simulink model "Nanogrid"  (R2026a)
settings: Solver=VariableStepAuto  StopTime=3
PreLoadFcn:
  | NanogridParam
undefined symbols (not defined in the file): baseLoad, bessSystem, bessVoltage, DiscIntNeverNeededParam, ee_sli_rtmsupport, gcbh, gflInverter, gfmInverter, nanoLoad, PV, PVInverter, ref, solar, solarInsolationChange, Ts
libraries: nesl_utility x51, eeGeneralControl x38, ee_lib x33, fl_lib x24, simulink x20, eeTransforms x13, slpidlib x8, nesl_utility_internal x4, sl_signal_attributes x4, sl_discontinuities x4, eeSinusoidalMeasurementV2 x3, batteryecm_lib x2
(part 6 of 6)

== system Nanogrid/Solar Plant Integrated/Detailed/PV Plant & Controller/Controller/MPPT/Solar PV Controller/Variant Subsystem/P&O MPP ==
  Ipv : Inport
  Vpv : Inport  Port=2
  AND1 : Logic  IconShape=distinctive  AllPortsSameDT=off  OutDataTypeStr=boolean
  Add : Sum
  Compare To Zero1 : simulink/Logic and Bit Operations/Compare To Zero  relop=>=  OutDataTypeStr=boolean
  Compare To Zero2 : simulink/Logic and Bit Operations/Compare To Zero  relop=>=  OutDataTypeStr=boolean
  Constant1 : Constant  Value=delV  SampleTime=sampleTime
  Data Type Conversion Inherited : sl_signal_attributes/Data Type Conversion Inherited  ConvertRealWorld=Real World Value  DoSatur=off
  Data Type Conversion Inherited1 : sl_signal_attributes/Data Type Conversion Inherited  ConvertRealWorld=Real World Value  DoSatur=off
  Filtered Derivative (Discrete or Continuous) : eeGeneralControl/Filtered Derivative (Discrete or Continuous)  K=1  T=tSettling*2  B=inf  A=-inf  minRatio=1  init_option=Inherited from block input  x0=0  Ts=sampleTime
  Filtered Derivative (Discrete or Continuous)1 : eeGeneralControl/Filtered Derivative (Discrete or Continuous)  K=1  T=tSettling*2  B=inf  A=-inf  minRatio=1  init_option=Inherited from block input  x0=0  Ts=sampleTime
  NOR : Logic  Operator=NOR  IconShape=distinctive  AllPortsSameDT=off  OutDataTypeStr=boolean
  OR : Logic  Operator=OR  IconShape=distinctive  AllPortsSameDT=off  OutDataTypeStr=boolean
  Product : Product
  Subtract5 : Sum  Inputs=-+
  Switch4 : Switch  Criteria=u2 ~= 0  SaturateOnIntegerOverflow=off  InputSameDT=off
  Switch5 : Switch  Criteria=u2 > Threshold  SaturateOnIntegerOverflow=off  InputSameDT=off
  start MPPT Voltage : Constant  Value=Vdc  SampleTime=sampleTime
  Vmpp : Outport  VectorParamsAs1DForOutWhenUnconnected=off
  wires:
  Data Type Conversion Inherited1/1 -> Subtract5/1, Add/2
  start MPPT Voltage/1 -> Data Type Conversion Inherited/2
  Data Type Conversion Inherited/1 -> Switch5/3
  Switch4/1 -> Vmpp/1
  Product/1 -> Filtered Derivative (Discrete or Continuous)/1
  Ipv/1 -> Product/1
  [Vinc] -> Switch4/1
  AND1/1 -> OR/1
  Filtered Derivative (Discrete or Continuous)/1 -> Compare To Zero2/1
  Filtered Derivative (Discrete or Continuous)1/1 -> Compare To Zero1/1
  [Vdec] -> Switch4/3
  Subtract5/1 -> [Vdec]  "DEC"
  NOR/1 -> OR/2
  Add/1 -> [Vinc]  "INC"
  Vpv/1 -> Switch5/1, Switch5/2, Data Type Conversion Inherited/1, Filtered Derivative (Discrete or Continuous)1/1, Product/2
  Constant1/1 -> Data Type Conversion Inherited1/2
  Switch5/1 -> Subtract5/2, Add/1, Data Type Conversion Inherited1/1
  Compare To Zero2/1 -> AND1/1, NOR/2
  Compare To Zero1/1 -> AND1/2, NOR/1
  OR/1 -> Switch4/2

== system Nanogrid/Solar Plant Integrated/Detailed/PV Plant & Controller/Controller/Power Reference/Power Reference Controller/PLL & Measurements/Measurement1 ==
  u : Inport
  Lead-Lag (Discrete or Continuous) : eeGeneralControl/Lead-Lag (Discrete or Continuous)  T1=0  T2=1e-3  B=inf  A=-inf  init_option=Inherited from block input  x0=0  Ts=Ts
  Vg : Outport
  wires:
  u/1 -> Lead-Lag (Discrete or Continuous)/1
  Lead-Lag (Discrete or Continuous)/1 -> Vg/1

== system Nanogrid/Solar Plant Integrated/Detailed/PV Plant & Controller/Controller/Power Reference/Power Reference Controller/PLL & Measurements/Measurement2 ==
  u : Inport
  Lead-Lag (Discrete or Continuous) : eeGeneralControl/Lead-Lag (Discrete or Continuous)  T1=0  T2=1e-3  B=inf  A=-inf  init_option=Inherited from block input  x0=0  Ts=Ts
  Vg : Outport
  wires:
  u/1 -> Lead-Lag (Discrete or Continuous)/1
  Lead-Lag (Discrete or Continuous)/1 -> Vg/1

== system Nanogrid/Solar Plant Integrated/Detailed/PV Plant & Controller/Controller/Power Reference/Power Reference Controller/PLL & Measurements/Subsystem ==
  Vabc : Inport
  Iabc : Inport  Port=2
  Demux : Demux  Outputs=3
  Demux1 : Demux  Outputs=3
  Park Transform : eeTransforms/Park Transform  AxisAlignment=Q-axis  PowerInvariant=off
  Park Transform1 : eeTransforms/Park Transform  AxisAlignment=Q-axis  PowerInvariant=off
  Scope : Scope  NumInputPorts=2
      settings: ActiveDisplayYMinimum=0.97158  ActiveDisplayYMaximum=1.00612  DataLoggingVariableName=ScopeData5
  "Sinusoidal Measurement (PLL, Three-Phase)" : eeSinusoidalMeasurementV2/Sinusoidal Measurement (PLL, Three-Phase)  InputFilter=on  InputNormalization=off  Kp_LF=kpPLL  Ki_LF=kiPLL  F0=frequency  Theta0=0  Ts=-1
  Terminator : Terminator
  Terminator1 : Terminator
  mag : Outport
  freq : Outport  Port=2
  angle : Outport  Port=3
  Vd : Outport  Port=4
  Vq : Outport  Port=5
  Id1 : Outport  Port=6
  Iq1 : Outport  Port=7
  wires:
  Iabc/1 -> Park Transform1/1
  Demux1/3 -> Terminator1/1
  Demux1/2 -> Iq1/1
  Demux1/1 -> Id1/1
  Park Transform1/1 -> Demux1/1
  "Sinusoidal Measurement (PLL, Three-Phase)"/3 -> mag/1
  "Sinusoidal Measurement (PLL, Three-Phase)"/1 -> freq/1
  "Sinusoidal Measurement (PLL, Three-Phase)"/2 -> Park Transform/2, Park Transform1/2, angle/1
  Demux/2 -> Vq/1, Scope/2
  Demux/1 -> Vd/1, Scope/1
  Park Transform/1 -> Demux/1
  Vabc/1 -> "Sinusoidal Measurement (PLL, Three-Phase)"/1, Park Transform/1
  Demux/3 -> Terminator/1

== system Nanogrid/Solar Plant Integrated/Detailed/PV Plant & Controller/Controller/Power Reference/Power Reference Controller/Power Reference Controller/Current_controller ==
  id-ref : Inport
  ipvd : Inport  Port=2
  iqref : Inport  Port=3
  iq : Inport  Port=4
  Vd : Inport  Port=5
  Vq : Inport  Port=6
  Constant4 : Constant  Value=0
  Gain1 : Gain  Gain=2*1*pi*60*L/zbase
  Gain2 : Gain  Gain=2*1*pi*60*L/zbase
  Mux1 : Mux  Inputs=3
  PID Controller : slpidlib/PID Controller  Controller=PID  Form=Parallel  TimeDomain=Discrete-time  UseExternalTs=off  SampleTime=-1  IntegratorMethod=Forward Euler  FilterMethod=Forward Euler  ControllerParametersSource=internal  P=Kpic  I=Kiic  UseKiTs=off  D=Kd  UseExternalDerivativeSource=off  N=100  UseFilter=on  TunerSelectOption=Transfer Function Based (PID Tuner App)  InitialConditionSource=internal  InitialConditionForIntegrator=0  InitialConditionForFilter=0  DifferentiatorICPrevScaledInput=0  ExternalReset=none  TrackingMode=off  Kt=1  LimitOutput=on  SatLimitsSource=internal  UpperSaturationLimit=3  LowerSaturationLimit=-3  LinearizeAsGain=on  AntiWindupMode=clamping  Kb=1  LimitIntegrator=on  UpperIntegratorSaturationLimit=3  LowerIntegratorSaturationLimit=-3  POutMin=[]  POutMax=[]  IOutMin=[]  IOutMax=[]  DOutMin=[]  DOutMax=[]  NOutMin=[]  NOutMax=[]  SumOutMin=[]  SumOutMax=[]  SaturationOutMin=[]  SaturationOutMax=[]  PParamMin=[]  PParamMax=[]  IParamMin=[]  IParamMax=[]  DParamMin=[]  DParamMax=[]  NParamMin=[]  NParamMax=[]  KbParamMin=[]  KbParamMax=[]  KtParamMin=[]  KtParamMax=[]  KbOutMin=[]  KbOutMax=[]  KtOutMin=[]  KtOutMax=[]  IntegratorOutMin=[]  IntegratorOutMax=[]  FilterOutMin=[]  FilterOutMax=[]  SumI1OutMin=[]  SumI1OutMax=[]  SumI2OutMin=[]  SumI2OutMax=[]  SumI3OutMin=[]  SumI3OutMax=[]  SumI4OutMin=[]  SumI4OutMax=[]  SumDOutMin=[]  SumDOutMax=[]  DifferentiatorOutMin=[]  DifferentiatorOutMax=[]  FilterDiffOutCoefMin=[]  FilterDiffOutCoefMax=[]  ReciprocalOutMin=[]  ReciprocalOutMax=[]  SumDenOutMin=[]  SumDenOutMax=[]  SumNumOutMin=[]  SumNumOutMax=[]  DivideOutMin=[]  DivideOutMax=[]  UdiffTsProdOutMin=[]  UdiffTsProdOutMax=[]  NTsProdOutMin=[]  NTsProdOutMax=[]  UintegralTsProdOutMin=[]  UintegralTsProdOutMax=[]  UngainTsProdOutMin=[]  UngainTsProdOutMax=[]  ClampingZeroOutDataTypeStr=Inherit: Inherit via back propagation  ClampingZeroOutMin=[]  ClampingZeroOutMax=[]  FilterDenConstantOutDataTypeStr=Inherit: Inherit via back propagation  FilterDenConstantOutMin=[]  FilterDenConstantOutMax=[]  PCopyOutDataTypeStr=Inherit: Inherit via back propagation  PCopyOutMin=[]  PCopyOutMax=[]  NCopyOutDataTypeStr=Inherit: Inherit via back propagation  NCopyOutMin=[]  NCopyOutMax=[]  IntegratorContinuousStateAttributes=''  IntegratorStateMustResolveToSignalObject=off  IntegratorRTWStateStorageClass=Auto  FilterContinuousStateAttributes=''  FilterStateMustResolveToSignalObject=off  FilterRTWStateStorageClass=Auto  ParallelPVariant=InternalParameters  IdealPVariant=Disabled  IVariant=InternalParameters  DVariant=InternalParameters  IntegratorVariant=Discrete  SatVariant=Enabled  AWVariant=DiscClampingParallel  PCopyVariant=Disabled  TRVariant=Disabled  FdbkBlocksVariant=Forward  IdealPFdbkVariant=Disabled  SatFdbkVariant=Disabled  DerivativeFilterVariant=ForwardEulerFilter  NVariant=InternalParameters  NCopyVariant=Disabled  FilterICVariant=InternalICsFilter  IntegratorICVariant=InternalICs  ExternalResetVariant=Disabled  TRSumVariant=Passthrough  SumFdbkVariant=Disabled  SumVariant=Sum_PID  TsampFilterVariant=InternalTs  TsampNgainVariant=Passthrough  TsampIntegralVariant=Disabled_SignalSpec  ExternalSaturationOutDataTypeStr=Inherit: Same as second input  DerivativeSourceVariant=ErrorSignal  PreIntVariant=InternalPreInt
  PID Controller1 : slpidlib/PID Controller  Controller=PID  Form=Parallel  TimeDomain=Discrete-time  UseExternalTs=off  SampleTime=-1  IntegratorMethod=Forward Euler  FilterMethod=Forward Euler  ControllerParametersSource=internal  P=Kpic  I=Kiic  UseKiTs=off  D=Kd  UseExternalDerivativeSource=off  N=100  UseFilter=on  TunerSelectOption=Transfer Function Based (PID Tuner App)  InitialConditionSource=internal  InitialConditionForIntegrator=0  InitialConditionForFilter=0  DifferentiatorICPrevScaledInput=0  ExternalReset=none  TrackingMode=off  Kt=1  LimitOutput=on  SatLimitsSource=internal  UpperSaturationLimit=3  LowerSaturationLimit=-3  LinearizeAsGain=on  AntiWindupMode=clamping  Kb=1  LimitIntegrator=on  UpperIntegratorSaturationLimit=3  LowerIntegratorSaturationLimit=-3  POutMin=[]  POutMax=[]  IOutMin=[]  IOutMax=[]  DOutMin=[]  DOutMax=[]  NOutMin=[]  NOutMax=[]  SumOutMin=[]  SumOutMax=[]  SaturationOutMin=[]  SaturationOutMax=[]  PParamMin=[]  PParamMax=[]  IParamMin=[]  IParamMax=[]  DParamMin=[]  DParamMax=[]  NParamMin=[]  NParamMax=[]  KbParamMin=[]  KbParamMax=[]  KtParamMin=[]  KtParamMax=[]  KbOutMin=[]  KbOutMax=[]  KtOutMin=[]  KtOutMax=[]  IntegratorOutMin=[]  IntegratorOutMax=[]  FilterOutMin=[]  FilterOutMax=[]  SumI1OutMin=[]  SumI1OutMax=[]  SumI2OutMin=[]  SumI2OutMax=[]  SumI3OutMin=[]  SumI3OutMax=[]  SumI4OutMin=[]  SumI4OutMax=[]  SumDOutMin=[]  SumDOutMax=[]  DifferentiatorOutMin=[]  DifferentiatorOutMax=[]  FilterDiffOutCoefMin=[]  FilterDiffOutCoefMax=[]  ReciprocalOutMin=[]  ReciprocalOutMax=[]  SumDenOutMin=[]  SumDenOutMax=[]  SumNumOutMin=[]  SumNumOutMax=[]  DivideOutMin=[]  DivideOutMax=[]  UdiffTsProdOutMin=[]  UdiffTsProdOutMax=[]  NTsProdOutMin=[]  NTsProdOutMax=[]  UintegralTsProdOutMin=[]  UintegralTsProdOutMax=[]  UngainTsProdOutMin=[]  UngainTsProdOutMax=[]  ClampingZeroOutDataTypeStr=Inherit: Inherit via back propagation  ClampingZeroOutMin=[]  ClampingZeroOutMax=[]  FilterDenConstantOutDataTypeStr=Inherit: Inherit via back propagation  FilterDenConstantOutMin=[]  FilterDenConstantOutMax=[]  PCopyOutDataTypeStr=Inherit: Inherit via back propagation  PCopyOutMin=[]  PCopyOutMax=[]  NCopyOutDataTypeStr=Inherit: Inherit via back propagation  NCopyOutMin=[]  NCopyOutMax=[]  IntegratorContinuousStateAttributes=''  IntegratorStateMustResolveToSignalObject=off  IntegratorRTWStateStorageClass=Auto  FilterContinuousStateAttributes=''  FilterStateMustResolveToSignalObject=off  FilterRTWStateStorageClass=Auto  ParallelPVariant=InternalParameters  IdealPVariant=Disabled  IVariant=InternalParameters  DVariant=InternalParameters  IntegratorVariant=Discrete  SatVariant=Enabled  AWVariant=DiscClampingParallel  PCopyVariant=Disabled  TRVariant=Disabled  FdbkBlocksVariant=Forward  IdealPFdbkVariant=Disabled  SatFdbkVariant=Disabled  DerivativeFilterVariant=ForwardEulerFilter  NVariant=InternalParameters  NCopyVariant=Disabled  FilterICVariant=InternalICsFilter  IntegratorICVariant=InternalICs  ExternalResetVariant=Disabled  TRSumVariant=Passthrough  SumFdbkVariant=Disabled  SumVariant=Sum_PID  TsampFilterVariant=InternalTs  TsampNgainVariant=Passthrough  TsampIntegralVariant=Disabled_SignalSpec  ExternalSaturationOutDataTypeStr=Inherit: Same as second input  DerivativeSourceVariant=ErrorSignal  PreIntVariant=InternalPreInt
  Saturation : Saturate  UpperLimit=1.2  LowerLimit=-1.2
  Saturation1 : Saturate  UpperLimit=1.2  LowerLimit=-1.2
  Scope : Scope  NumInputPorts=2
      settings: ActiveDisplayYMinimum=0.49995  ActiveDisplayYMaximum=0.50039
  Scope1 : Scope  NumInputPorts=2
      settings: ActiveDisplayYMinimum=-1  ActiveDisplayYMaximum=1  DataLoggingVariableName=ScopeData2
  Scope2 : Scope  NumInputPorts=3
      settings: ActiveDisplayYMinimum=0.92426  ActiveDisplayYMaximum=1.0261  DataLoggingVariableName=ScopeData2
  Sum1 : Sum  Inputs=|+-
  Sum3 : Sum  Inputs=|++-
  Sum4 : Sum  Inputs=|+++
  Sum5 : Sum  Inputs=|+-
  mdq0 : Outport
  wires:
  Vd/1 -> Sum3/1, Scope2/1
  Saturation1/1 -> Mux1/2
  Saturation/1 -> Mux1/1
  iqref/1 -> Sum5/1, Scope1/1
  Mux1/1 -> mdq0/1
  Sum4/1 -> [Eq], Saturation1/1
  PID Controller1/1 -> Sum4/1
  Sum5/1 -> PID Controller1/1
  Constant4/1 -> Mux1/3
  Sum1/1 -> PID Controller/1
  iq/1 -> Sum5/2, Gain2/1, Scope1/2
  Vq/1 -> Sum4/2
  Gain1/1 -> Sum4/3
  id-ref/1 -> Sum1/1, Scope/1
  ipvd/1 -> Sum1/2, Gain1/1, Scope/2
  Gain2/1 -> Sum3/3, Scope2/3
  Sum3/1 -> [Ed], Saturation/1
  PID Controller/1 -> Sum3/2, Scope2/2

== system Nanogrid/Solar Plant Integrated/Detailed/PV Plant & Controller/Controller/Power Reference/Power Reference Controller/Power Reference Controller/Reference Current ==
  note: Avoid division by zero during start
  note: Current Limiters
  V-mag : Inport
  LVRT_iq : Inport  Port=2
  PRef : Inport  Port=3
  QRef : Inport  Port=4
  Constant1 : Constant
  Constant3 : Constant  Value=Imax
  Current limits : Subsystem
  Refernce id generation : Subsystem
  Refernce iq generation : Subsystem
  Switch : Switch  Criteria=u2 ~= 0  SaturateOnIntegerOverflow=off  InputSameDT=off
  Unit Delay1 : UnitDelay  SampleTime=Ts
  Unit Delay3 : UnitDelay  SampleTime=Ts
  id_ref : Outport
  iq_ref : Outport  Port=2
  wires:
  Current limits/2(iubd) -> Refernce id generation/2(ubid)
  PRef/1 -> Refernce id generation/3(PRef)
  QRef/1 -> Refernce iq generation/4(Q_ref)
  Constant1/1 -> Switch/3
  Switch/1 -> Refernce iq generation/2(V_mag), Refernce id generation/1(V_mag)
  V-mag/1 -> Switch/2, Switch/1
  LVRT_iq/1 -> Refernce iq generation/3(LVRT_iq)
  Refernce iq generation/1(iq_ref) -> iq_ref/1, Unit Delay1/1
  Refernce id generation/1(id_ref) -> Unit Delay3/1, id_ref/1
  Constant3/1 -> Current limits/1(Imax)
  Unit Delay3/1 -> Current limits/3(idref)
  Current limits/1(iubq) -> Refernce iq generation/1(ubiq)
  Unit Delay1/1 -> Current limits/2(iqref)

== system Nanogrid/BESS Integrated/Detailed/BESS Controller/Grid Forming/Current Limiting/CurrentLimitingMethod/currentLimitAndVirtual/Current Saturation/Compare ==
  u : Inport
  Compare To Zero : simulink/Logic and Bit Operations/Compare To Zero  relop=<=  OutDataTypeStr=boolean
  Data Type Conversion : DataTypeConversion  SaturateOnIntegerOverflow=off  RndMeth=Floor
  Out1 : Outport
  wires:
  Data Type Conversion/1 -> Out1/1
  u/1 -> Compare To Zero/1
  Compare To Zero/1 -> Data Type Conversion/1

== system Nanogrid/BESS Integrated/Detailed/BESS Controller/Grid Forming/Current Limiting/CurrentLimitingMethod/currentLimitAndVirtual/Current Saturation/If Action Subsystem ==
  Is : Inport
  Isd : Inport  Port=2
  Isq : Inport  Port=3
  maxI : Inport  Port=4
  Action Port : ActionPort
  Divide : Product  Inputs=*/
  Product : Product
  Product1 : Product
  Idmax : Outport
  Iqmax : Outport  Port=2
  wires:
  Product/1 -> Iqmax/1
  Product1/1 -> Idmax/1
  Isq/1 -> Product/2
  Isd/1 -> Product1/1
  Divide/1 -> Product/1, Product1/2
  Is/1 -> Divide/2
  maxI/1 -> Divide/1

== system Nanogrid/BESS Integrated/Detailed/BESS Controller/Grid Forming/Current Limiting/CurrentLimitingMethod/currentLimitAndVirtual/Current Saturation/If Action Subsystem1 ==
  Action Port : ActionPort
  Constant3 : Constant  Value=0
  Constant4 : Constant  Value=0
  Idmax : Outport
  Iqmax : Outport  Port=2
  wires:
  Constant3/1 -> Idmax/1
  Constant4/1 -> Iqmax/1

== system Nanogrid/BESS Integrated/Detailed/BESS Controller/Grid Forming/Measurement/Frequency Measurement/Frequency Measurement/If Action Subsystem/Frequency estimation ==
  sk : Inport
  sk-1 : Inport  Port=2
  k : Inport  Port=3
  k-1 : Inport  Port=4
  Trigger : TriggerPort  VariantControl=(inherit)  InitialTriggerSignalState=positive
  Add1 : Sum  Inputs=+-  OutDataTypeStr=double  AccumDataTypeStr=double  RndMeth=Convergent
  Add2 : Sum
  Constant : Constant
  Delay : Delay  DelayLength=1
  Delay1 : Delay  DelayLength=1
  Divide : Product  Inputs=*/  RndMeth=Ceiling
  Gain : Gain  Gain=2  ParamDataTypeStr=double  RndMeth=Convergent
  Gain2 : Gain  Gain=0.5
  MATLAB Function : MATLAB Function  TreatAsAtomicUnit=on
  f : Outport
  wires:
  sk-1/1 -> MATLAB Function/2(y2)
  sk/1 -> MATLAB Function/1(y1)
  k-1/1 -> MATLAB Function/4(x2)  "x1"
  k/1 -> MATLAB Function/3(x1)
  Delay/1 -> Add1/2
  Gain2/1 -> f/1
  Add2/1 -> Gain2/1
  Delay1/1 -> Add2/2
  Divide/1 -> Delay1/1, Add2/1
  MATLAB Function/1(x) -> Add1/1, Delay/1  "x1-y1/slope"
  Gain/1 -> Divide/2
  Constant/1 -> Divide/1
  Add1/1 -> Gain/1

== system Nanogrid/BESS Integrated/Detailed/BESS Controller/Grid Forming/Power Control/ActivePowerControl/vsmControl/Damping Frequency/ConstantFreqReference ==
  fref : Inport
  Constant1 : Constant
  Terminator : Terminator
  fmeas : Outport
  wires:
  fref/1 -> Terminator/1
  Constant1/1 -> fmeas/1

== system Nanogrid/BESS Integrated/Detailed/BESS Controller/Grid Forming/Power Control/ActivePowerControl/vsmControl/Damping Frequency/WithFrequencyMeasurement ==
  fref : Inport
  fmeas : Outport
  wires:
  fref/1 -> fmeas/1

== system Nanogrid/BESS Integrated/Detailed/BESS Controller/Grid Forming/Power Control/ActivePowerControl/vsmControl/Power Reference Selection/If Action Subsystem ==
  note: Frequency difference power
  Pref : Inport
  Wsm : Inport  Port=2
  Action Port : ActionPort  ActionPortLabel=if(u1 > 0)
  Constant : Constant
  Gain6 : Gain  Gain=vsmFreqDroop
  Sum : Sum  Inputs=|+-
  Sum3 : Sum  Inputs=++|
  Power : Outport
  wires:
  Sum3/1 -> Power/1
  Constant/1 -> Sum/1
  Sum/1 -> Gain6/1
  Wsm/1 -> Sum/2
  Pref/1 -> Sum3/1  "Reference power"
  Gain6/1 -> Sum3/2

== system Nanogrid/BESS Integrated/Detailed/BESS Controller/Grid Forming/Power Control/ActivePowerControl/vsmControl/Power Reference Selection/If Action Subsystem1 ==
  note: Frequency difference power
  fref : Inport
  Wsm : Inport  Port=2
  Action Port : ActionPort  ActionPortLabel=else
  Gain6 : Gain  Gain=vsmFreqDroop
  Scope : Scope
      settings: ActiveDisplayYMinimum=0.99966  ActiveDisplayYMaximum=1.00057  DataLoggingVariableName=ScopeData14
  Scope1 : Scope
      settings: DataLoggingVariableName=ScopeData15
  Sum : Sum  Inputs=|+-
  Power : Outport
  wires:
  Gain6/1 -> Power/1, Scope1/1
  fref/1 -> Sum/1
  Sum/1 -> Gain6/1
  Wsm/1 -> Sum/2, Scope/1

== system Nanogrid/Solar Plant Integrated/Detailed/PV Plant & Controller/Controller/MPPT/Solar PV Controller/DC voltage controller & current reference/If Action Subsystem/Subsystem ==
  V mag : Inport
  iq ub : Inport  Port=2
  Q ref : Inport  Port=3
  Constant : Constant  Value=1e-3
  Data Type Conversion Inherited : simulink/Signal Attributes/Data Type Conversion Inherited  ConvertRealWorld=Real World Value  DoSatur=off
  Divide2 : Product  Inputs=*/
  Gain3 : Gain  Gain=-1
  Saturation Dynamic2 : simulink/Discontinuities/Saturation Dynamic  OutMin=[]  OutMax=[]  OutDataTypeStr=Inherit: Same as second input  OutDataType=fixdt(1, 16)  OutScaling=2^-10  DoSatur=off
  Switch : Switch  Criteria=u2 ~= 0  SaturateOnIntegerOverflow=off  InputSameDT=off
  iq ub1 : InportShadow  Port=2
  iqref : Outport
  wires:
  Data Type Conversion Inherited/1 -> Switch/3
  Constant/1 -> Data Type Conversion Inherited/2
  Switch/1 -> Divide2/2
  V mag/1 -> Switch/1, Switch/2, Data Type Conversion Inherited/1
  Saturation Dynamic2/1 -> iqref/1
  iq ub/1 -> Saturation Dynamic2/1
  Gain3/1 -> Saturation Dynamic2/3
  Q ref/1 -> Divide2/1
  Divide2/1 -> Saturation Dynamic2/2
  iq ub1/1 -> Gain3/1

== system Nanogrid/Solar Plant Integrated/Detailed/PV Plant & Controller/Controller/MPPT/Solar PV Controller/DC voltage controller & current reference/If Action Subsystem/Subsystem1 ==
  Vmag : Inport
  P pv : Inport  Port=2
  vdc : Inport  Port=3
  vdc ref : Inport  Port=4
  id ub : Inport  Port=5
  Constant : Constant  Value=1e-3
  Constant4 : Constant  Value=0
  Data Type Conversion Inherited : simulink/Signal Attributes/Data Type Conversion Inherited  ConvertRealWorld=Real World Value  DoSatur=off
  Divide : Product  Inputs=/*
  Gain4 : Gain  Gain=1/(mVAbase)
  Saturation Dynamic1 : simulink/Discontinuities/Saturation Dynamic  OutMin=[]  OutMax=[]  OutDataTypeStr=Inherit: Same as second input  OutDataType=fixdt(1, 16)  OutScaling=2^-10  DoSatur=off
  Scope : Scope  NumInputPorts=2
      settings: ActiveDisplayYMinimum=-55957.97767  ActiveDisplayYMaximum=503630.2665
  Sum : Sum  Inputs=|++
  Switch : Switch  Criteria=u2 ~= 0  SaturateOnIntegerOverflow=off  InputSameDT=off
  V_dc_Controller1 : Subsystem
  idref : Outport
  wires:
  Data Type Conversion Inherited/1 -> Switch/3
  Constant/1 -> Data Type Conversion Inherited/2
  Switch/1 -> Divide/1
  Vmag/1 -> Switch/1, Switch/2, Data Type Conversion Inherited/1
  vdc/1 -> Scope/1, V_dc_Controller1/1(vdc)
  Saturation Dynamic1/1 -> idref/1
  Divide/1 -> Sum/1
  Gain4/1 -> Divide/2
  id ub/1 -> Saturation Dynamic1/1
  vdc ref/1 -> Scope/2, V_dc_Controller1/2(vdc ref)
  Sum/1 -> Saturation Dynamic1/2
  V_dc_Controller1/1(Out1) -> Sum/2
  P pv/1 -> Gain4/1
  Constant4/1 -> Saturation Dynamic1/3

== system Nanogrid/Solar Plant Integrated/Detailed/PV Plant & Controller/Controller/MPPT/Solar PV Controller/DC voltage controller & current reference/Subsystem1/V_dc_Controller1 ==
  vdc : Inport
  vdc ref : Inport  Port=2
  Gain : Gain  Gain=1/VdcBase
  PID Controller : slpidlib/PID Controller  Controller=PID  Form=Parallel  TimeDomain=Discrete-time  UseExternalTs=off  SampleTime=-1  IntegratorMethod=Forward Euler  FilterMethod=Forward Euler  ControllerParametersSource=internal  P=Kpv  I=Kiv  UseKiTs=off  D=Kdv  UseExternalDerivativeSource=off  N=100  UseFilter=on  TunerSelectOption=Transfer Function Based (PID Tuner App)  ZeroCross=off  InitialConditionSource=internal  InitialConditionForIntegrator=0  InitialConditionForFilter=0  DifferentiatorICPrevScaledInput=0  ExternalReset=none  TrackingMode=off  Kt=1  LimitOutput=off  SatLimitsSource=internal  UpperSaturationLimit=iMax  LowerSaturationLimit=0  LinearizeAsGain=on  AntiWindupMode=clamping  Kb=1  LimitIntegrator=off  UpperIntegratorSaturationLimit=inf  LowerIntegratorSaturationLimit=-inf  POutMin=[]  POutMax=[]  IOutMin=[]  IOutMax=[]  DOutMin=[]  DOutMax=[]  NOutMin=[]  NOutMax=[]  SumOutMin=[]  SumOutMax=[]  SaturationOutMin=[]  SaturationOutMax=[]  PParamMin=[]  PParamMax=[]  IParamMin=[]  IParamMax=[]  DParamMin=[]  DParamMax=[]  NParamMin=[]  NParamMax=[]  KbParamMin=[]  KbParamMax=[]  KtParamMin=[]  KtParamMax=[]  KbOutMin=[]  KbOutMax=[]  KtOutMin=[]  KtOutMax=[]  IntegratorOutMin=[]  IntegratorOutMax=[]  FilterOutMin=[]  FilterOutMax=[]  SumI1OutMin=[]  SumI1OutMax=[]  SumI2OutMin=[]  SumI2OutMax=[]  SumI3OutMin=[]  SumI3OutMax=[]  SumI4OutMin=[]  SumI4OutMax=[]  SumDOutMin=[]  SumDOutMax=[]  DifferentiatorOutMin=[]  DifferentiatorOutMax=[]  FilterDiffOutCoefMin=[]  FilterDiffOutCoefMax=[]  ReciprocalOutMin=[]  ReciprocalOutMax=[]  SumDenOutMin=[]  SumDenOutMax=[]  SumNumOutMin=[]  SumNumOutMax=[]  DivideOutMin=[]  DivideOutMax=[]  UdiffTsProdOutMin=[]  UdiffTsProdOutMax=[]  NTsProdOutMin=[]  NTsProdOutMax=[]  UintegralTsProdOutMin=[]  UintegralTsProdOutMax=[]  UngainTsProdOutMin=[]  UngainTsProdOutMax=[]  ClampingZeroOutDataTypeStr=Inherit: Inherit via back propagation  ClampingZeroOutMin=[]  ClampingZeroOutMax=[]  FilterDenConstantOutDataTypeStr=Inherit: Inherit via back propagation  FilterDenConstantOutMin=[]  FilterDenConstantOutMax=[]  PCopyOutDataTypeStr=Inherit: Inherit via back propagation  PCopyOutMin=[]  PCopyOutMax=[]  NCopyOutDataTypeStr=Inherit: Inherit via back propagation  NCopyOutMin=[]  NCopyOutMax=[]  IntegratorContinuousStateAttributes=''  IntegratorStateMustResolveToSignalObject=off  IntegratorRTWStateStorageClass=Auto  FilterContinuousStateAttributes=''  FilterStateMustResolveToSignalObject=off  FilterRTWStateStorageClass=Auto  ParallelPVariant=InternalParameters  IdealPVariant=Disabled  IVariant=InternalParameters  DVariant=InternalParameters  IntegratorVariant=Discrete  SatVariant=Disabled  AWVariant=Passthrough  PCopyVariant=Disabled  TRVariant=Disabled  FdbkBlocksVariant=Forward  IdealPFdbkVariant=Disabled  SatFdbkVariant=Disabled  DerivativeFilterVariant=ForwardEulerFilter  NVariant=InternalParameters  NCopyVariant=Disabled  FilterICVariant=InternalICsFilter  IntegratorICVariant=InternalICs  ExternalResetVariant=Disabled  TRSumVariant=Passthrough  SumFdbkVariant=Disabled  SumVariant=Sum_PID  TsampFilterVariant=InternalTs  TsampNgainVariant=Passthrough  TsampIntegralVariant=Disabled_SignalSpec  ExternalSaturationOutDataTypeStr=Inherit: Same as second input  DerivativeSourceVariant=ErrorSignal  PreIntVariant=InternalPreInt
  Sum : Sum  Inputs=|+-
  Out1 : Outport
  wires:
  Sum/1 -> Gain/1
  Gain/1 -> PID Controller/1
  PID Controller/1 -> Out1/1
  vdc ref/1 -> Sum/2
  vdc/1 -> Sum/1

== system Nanogrid/Solar Plant Integrated/Detailed/PV Plant & Controller/Controller/Power Reference/Power Reference Controller/Power Reference Controller/Reference Current/Current limits ==
  Imax : Inport
  iqref : Inport  Port=2
  idref : Inport  Port=3
  Constant8 : Constant  Value=0
  Constant9 : Constant  Value=0
  Scope : Scope
      settings: ActiveDisplayYMinimum=-0.15  ActiveDisplayYMaximum=1.35  DataLoggingVariableName=ScopeData3
  Scope1 : Scope
      settings: ActiveDisplayYMinimum=-0.08298  ActiveDisplayYMaximum=0.74678  DataLoggingVariableName=ScopeData4
  Sqrt : Sqrt
  Sqrt1 : Sqrt
  Square{1..4} (4 alike) : Math  Operator=square
  Step2 : Step  Time=0.01  SampleTime=Ts
  Step3 : Step  Time=0.01  SampleTime=Ts
  Sum6 : Sum  Inputs=|+-
  Sum9 : Sum  Inputs=|+-
  Switch1 : Switch  Threshold=.01  SaturateOnIntegerOverflow=off  InputSameDT=off
  Switch2 : Switch  Threshold=.01  SaturateOnIntegerOverflow=off  InputSameDT=off
  iubq : Outport
  iubd : Outport  Port=2
  wires:
  idref/1 -> Square4/1
  Sqrt1/1 -> iubq/1, Scope1/1
  Imax/1 -> Square1/1, Square3/1
  Sqrt/1 -> iubd/1, Scope/1
  Constant9/1 -> Switch2/3
  Square4/1 -> Sum9/2
  Constant8/1 -> Switch1/3
  Square2/1 -> Sum6/2
  Sum6/1 -> Switch1/1
  Square3/1 -> Sum9/1
  iqref/1 -> Square2/1
  Switch1/1 -> Sqrt/1
  Square1/1 -> Sum6/1
  Switch2/1 -> Sqrt1/1
  Step2/1 -> Switch1/2
  Step3/1 -> Switch2/2
  Sum9/1 -> Switch2/1

== system Nanogrid/Solar Plant Integrated/Detailed/PV Plant & Controller/Controller/Power Reference/Power Reference Controller/Power Reference Controller/Reference Current/Refernce id generation ==
  V_mag : Inport
  ubid : Inport  Port=2
  PRef : Inport  Port=3
  Divide : Product  Inputs=/*
  Gain6 : Gain  Gain=-1
  P/Q Priority : Switch  Criteria=u2 ~= 0  SaturateOnIntegerOverflow=off  InputSameDT=off
  Priority Mode : Constant  Value=P-2
  Saturation Dynamic2 : sl_discontinuities/Saturation Dynamic  OutMin=[]  OutMax=[]  OutDataTypeStr=Inherit: Same as second input  OutDataType=fixdt(1, 16)  OutScaling=2^-10  DoSatur=off
  Saturation1 : Saturate  UpperLimit=Imax  LowerLimit=-Imax
  Scope : Scope
      settings: ActiveDisplayYMinimum=0.99583  ActiveDisplayYMaximum=1.02853
  Scope1 : Scope
      settings: ActiveDisplayYMinimum=-0.12499  ActiveDisplayYMaximum=1.12489  DataLoggingVariableName=ScopeData2
  ubid1 : InportShadow  Port=2
  id_ref : Outport
  wires:
  Divide/1 -> Saturation1/1, Saturation Dynamic2/2
  V_mag/1 -> Divide/1
  P/Q Priority/1 -> id_ref/1, Scope/1
  ubid1/1 -> Gain6/1
  Saturation1/1 -> P/Q Priority/1
  Priority Mode/1 -> P/Q Priority/2
  Saturation Dynamic2/1 -> P/Q Priority/3, Scope1/1
  Gain6/1 -> Saturation Dynamic2/3
  ubid/1 -> Saturation Dynamic2/1
  PRef/1 -> Divide/2

== system Nanogrid/Solar Plant Integrated/Detailed/PV Plant & Controller/Controller/Power Reference/Power Reference Controller/Power Reference Controller/Reference Current/Refernce iq generation ==
  ubiq : Inport
  V_mag : Inport  Port=2
  LVRT_iq : Inport  Port=3
  Q_ref : Inport  Port=4
  Divide1 : Product  Inputs=*/
  Gain : Gain  Gain=-1
  Gain1 : Gain  Gain=-1
  Gain7 : Gain  Gain=-1
  LVRT Priority : Switch  Threshold=.9  SaturateOnIntegerOverflow=off  InputSameDT=off
  P/Q Priority : Switch  Criteria=u2 ~= 0  SaturateOnIntegerOverflow=off  InputSameDT=off
  Priority Mode : Constant  Value=P-2
  Saturation Dynamic : sl_discontinuities/Saturation Dynamic  OutMin=[]  OutMax=[]  OutDataTypeStr=Inherit: Same as second input  OutDataType=fixdt(1, 16)  OutScaling=2^-10  DoSatur=off
  Saturation2 : Saturate  UpperLimit=1  LowerLimit=-1
  Saturation3 : Saturate  UpperLimit=Imax  LowerLimit=-Imax
  Scope : Scope  NumInputPorts=3
      settings: ActiveDisplayYMinimum=-0.025  ActiveDisplayYMaximum=0.22499  DataLoggingVariableName=ScopeData10
  ubiq1 : InportShadow
  iq_ref : Outport
  wires:
  Gain/1 -> iq_ref/1
  V_mag/1 -> Divide1/2, LVRT Priority/2
  Q_ref/1 -> Divide1/1
  ubiq1/1 -> Gain7/1
  LVRT_iq/1 -> Saturation2/1
  Gain7/1 -> Saturation Dynamic/3
  Saturation Dynamic/1 -> P/Q Priority/1
  Divide1/1 -> Saturation Dynamic/2, Saturation3/1
  Priority Mode/1 -> P/Q Priority/2
  Saturation3/1 -> P/Q Priority/3
  Saturation2/1 -> Gain1/1
  ubiq/1 -> Saturation Dynamic/1
  Gain1/1 -> LVRT Priority/3
  P/Q Priority/1 -> Scope/1, LVRT Priority/1
  LVRT Priority/1 -> Gain/1

== system Nanogrid/Solar Plant Integrated/Detailed/PV Plant & Controller/Controller/MPPT/Solar PV Controller/DC voltage controller & current reference/If Action Subsystem/Subsystem1/V_dc_Controller1 ==
  vdc : Inport
  vdc ref : Inport  Port=2
  Gain : Gain  Gain=1/VdcBase
  PID Controller : slpidlib/PID Controller  Controller=PID  Form=Parallel  TimeDomain=Discrete-time  UseExternalTs=off  SampleTime=-1  IntegratorMethod=Forward Euler  FilterMethod=Forward Euler  ControllerParametersSource=internal  P=Kpv  I=Kiv  UseKiTs=off  D=Kdv  UseExternalDerivativeSource=off  N=100  UseFilter=on  TunerSelectOption=Transfer Function Based (PID Tuner App)  ZeroCross=off  InitialConditionSource=internal  InitialConditionForIntegrator=0  InitialConditionForFilter=0  DifferentiatorICPrevScaledInput=0  ExternalReset=none  TrackingMode=off  Kt=1  LimitOutput=off  SatLimitsSource=internal  UpperSaturationLimit=iMax  LowerSaturationLimit=0  LinearizeAsGain=on  AntiWindupMode=clamping  Kb=1  LimitIntegrator=off  UpperIntegratorSaturationLimit=inf  LowerIntegratorSaturationLimit=-inf  POutMin=[]  POutMax=[]  IOutMin=[]  IOutMax=[]  DOutMin=[]  DOutMax=[]  NOutMin=[]  NOutMax=[]  SumOutMin=[]  SumOutMax=[]  SaturationOutMin=[]  SaturationOutMax=[]  PParamMin=[]  PParamMax=[]  IParamMin=[]  IParamMax=[]  DParamMin=[]  DParamMax=[]  NParamMin=[]  NParamMax=[]  KbParamMin=[]  KbParamMax=[]  KtParamMin=[]  KtParamMax=[]  KbOutMin=[]  KbOutMax=[]  KtOutMin=[]  KtOutMax=[]  IntegratorOutMin=[]  IntegratorOutMax=[]  FilterOutMin=[]  FilterOutMax=[]  SumI1OutMin=[]  SumI1OutMax=[]  SumI2OutMin=[]  SumI2OutMax=[]  SumI3OutMin=[]  SumI3OutMax=[]  SumI4OutMin=[]  SumI4OutMax=[]  SumDOutMin=[]  SumDOutMax=[]  DifferentiatorOutMin=[]  DifferentiatorOutMax=[]  FilterDiffOutCoefMin=[]  FilterDiffOutCoefMax=[]  ReciprocalOutMin=[]  ReciprocalOutMax=[]  SumDenOutMin=[]  SumDenOutMax=[]  SumNumOutMin=[]  SumNumOutMax=[]  DivideOutMin=[]  DivideOutMax=[]  UdiffTsProdOutMin=[]  UdiffTsProdOutMax=[]  NTsProdOutMin=[]  NTsProdOutMax=[]  UintegralTsProdOutMin=[]  UintegralTsProdOutMax=[]  UngainTsProdOutMin=[]  UngainTsProdOutMax=[]  ClampingZeroOutDataTypeStr=Inherit: Inherit via back propagation  ClampingZeroOutMin=[]  ClampingZeroOutMax=[]  FilterDenConstantOutDataTypeStr=Inherit: Inherit via back propagation  FilterDenConstantOutMin=[]  FilterDenConstantOutMax=[]  PCopyOutDataTypeStr=Inherit: Inherit via back propagation  PCopyOutMin=[]  PCopyOutMax=[]  NCopyOutDataTypeStr=Inherit: Inherit via back propagation  NCopyOutMin=[]  NCopyOutMax=[]  IntegratorContinuousStateAttributes=''  IntegratorStateMustResolveToSignalObject=off  IntegratorRTWStateStorageClass=Auto  FilterContinuousStateAttributes=''  FilterStateMustResolveToSignalObject=off  FilterRTWStateStorageClass=Auto  ParallelPVariant=InternalParameters  IdealPVariant=Disabled  IVariant=InternalParameters  DVariant=InternalParameters  IntegratorVariant=Discrete  SatVariant=Disabled  AWVariant=Passthrough  PCopyVariant=Disabled  TRVariant=Disabled  FdbkBlocksVariant=Forward  IdealPFdbkVariant=Disabled  SatFdbkVariant=Disabled  DerivativeFilterVariant=ForwardEulerFilter  NVariant=InternalParameters  NCopyVariant=Disabled  FilterICVariant=InternalICsFilter  IntegratorICVariant=InternalICs  ExternalResetVariant=Disabled  TRSumVariant=Passthrough  SumFdbkVariant=Disabled  SumVariant=Sum_PID  TsampFilterVariant=InternalTs  TsampNgainVariant=Passthrough  TsampIntegralVariant=Disabled_SignalSpec  ExternalSaturationOutDataTypeStr=Inherit: Same as second input  DerivativeSourceVariant=ErrorSignal  PreIntVariant=InternalPreInt
  Sum : Sum  Inputs=|+-
  Out1 : Outport
  wires:
  Sum/1 -> Gain/1
  Gain/1 -> PID Controller/1
  PID Controller/1 -> Out1/1
  vdc ref/1 -> Sum/2
  vdc/1 -> Sum/1

== stateflow chart Nanogrid/BESS Integrated/Detailed/BESS Controller/Grid Forming/Current Limiting/CurrentLimitingMethod/currentLimitAndVirtual/CurrentLimitSelection ==
  state Mode1_VI_ON
    entry:
    noCurrentLimit  = 0;
    viCurrentLimit = 1;
    satCurrentLimit = 0;
    ismax= maxVICurrentLimit;
    exit:
    noCurrentLimit  = 0;
    viCurrentLimit = 1;
    satCurrentLimit = 0;
    ismax= maxVICurrentLimit;
  state Start_Mode
    entry:
    noCurrentLimit  = 1;
    viCurrentLimit = 0;
    satCurrentLimit = 0;
    ismax= maxSatCurrentLimit;
    exit:
    noCurrentLimit  = 1;
    viCurrentLimit = 0;
    satCurrentLimit = 0;
    ismax= maxSatCurrentLimit;
  state Mode2_CurrentSat_ON
    entry:
    noCurrentLimit  = 0;
    viCurrentLimit = 0;
    satCurrentLimit = 1;
    ismax= maxSatCurrentLimit;
    exit:
    noCurrentLimit  = 0;
    viCurrentLimit = 0;
    satCurrentLimit = 1;
    ismax= maxSatCurrentLimit;
  state Mode3_CurrentSat_ON
    entry:
    noCurrentLimit  = 0;
    viCurrentLimit = 0;
    satCurrentLimit = 1;
    ismax= 1.1*maxVICurrentLimit;
    exit:
    noCurrentLimit  = 0;
    viCurrentLimit = 0;
    satCurrentLimit = 1;
    ismax= 1.1*maxVICurrentLimit;
  Start_Mode -> Mode1_VI_ON : [Is>1]
  (junction 28) -> Mode1_VI_ON : after(currentControlTs*10, sec)[(Is<ismax) && (Is>1) ]
  Mode3_CurrentSat_ON -> (junction 28) [order 1]
  (default) -> Start_Mode
  Mode1_VI_ON -> Start_Mode [order 2] : [Is<1]
  Mode1_VI_ON -> Mode2_CurrentSat_ON [order 1] : after(0.5/powerFreq, sec)[(Is>=maxSatCurrentLimit)]
  (junction 26) -> Start_Mode
  Mode3_CurrentSat_ON -> Mode2_CurrentSat_ON [order 2] : after(0.5/powerFreq, sec)[(Is>ismax)]
  Mode2_CurrentSat_ON -> Mode3_CurrentSat_ON : after(currentSatTime, sec)[satCurrentLimit>0]
  Mode3_CurrentSat_ON -> (junction 26) [order 3] : [Is<1]
  data: Is input; ismax output; noCurrentLimit output; viCurrentLimit output; satCurrentLimit output; maxSatCurrentLimit parameter; maxVICurrentLimit parameter; currentControlTs parameter; currentSatTime parameter; powerFreq parameter

== matlab function Nanogrid/BESS Integrated/Detailed/BESS Controller/Grid Forming/Measurement/Frequency Measurement/Frequency Measurement/If Action Subsystem/Frequency estimation/MATLAB Function ==
  data: y1 input; y2 input; x1 input; x output; x2 input
function x = fcn(y1,y2,x1,x2)
% Line equation between two points is y-y1=((y2-y1)/(x2-x1))*(x-x1). Here
% to to find the zero crossing instant substitute y = 0 and find x
slope = (y2-y1)/(x2-x1);
x = x1-y1/slope;
